simulink model "DS_SS"  (R2018a)
settings: Solver=ode4  StartTime=0.0  StopTime=N*Tb  FixedStep=Tsampling  RelTol=1e-9
values from neighbouring files (symbols this model uses):
  Eb = 2    [DS_Script.m]
  FrecSignal = MultFrec*(1/Tc)    [DS_MultUs_Script.m]    (also in DS_Script.m = 7500)
  Tb = 1/100    (= 0.01)    [DS_Script.m]
  Tc = Tb_min/(MultPer*Nchips)    [DS_MultUs_Script.m]    (also in DS_Script.m = 0.000666666666667)
libraries: commdigbbndpm3 x6, commseqgen3 x6, dspsigops x3, commutil2 x3, commrandsrc3 x3
settings Model: Creator=lukit  LastModifiedBy=geroo
settings DebuggingCC: LibraryContextMissingDiagnostic=warning
settings SFSimCC: SimUseLocalCustomCode=on
settings RTWCC: RTWUseLocalCustomCode=on

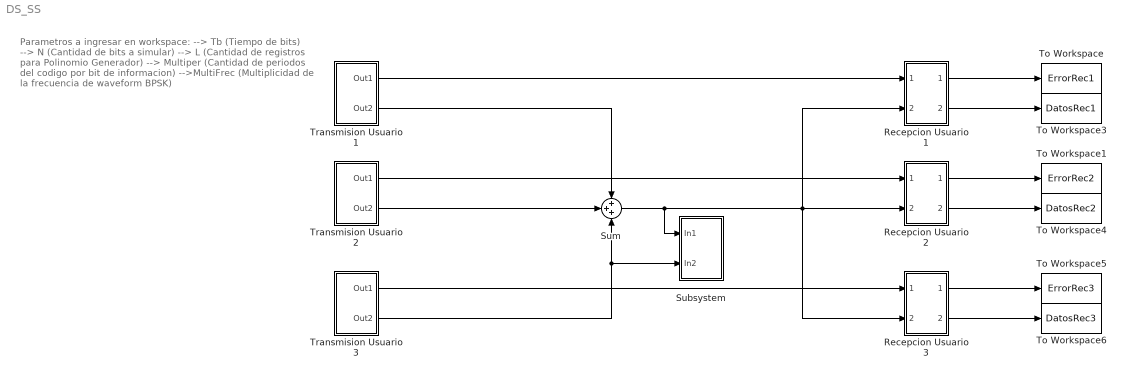
== system DS_SS ==
  note: Parametros a ingresar en workspace:
      | --> Tb (Tiempo de bits)
      | --> N  (Cantidad de bits a simular)
      | --> L   (Cantidad de registros para Polinomio Generador)
      | --> Multiper  (Cantidad de periodos del codigo por bit de informacion)
      | -->MultiFrec (Multiplicidad de la frecuencia de waveform BPSK)
  "Recepcion Usuario 1 " : Subsystem
  "Recepcion Usuario 2 " : Subsystem
  Recepcion Usuario 3 : Subsystem
  Subsystem : Subsystem
  Sum : Sum  Inputs=+++
  To Workspace : ToWorkspace  VariableName=ErrorRec1  SampleTime=-1
      settings: Save2DSignal=2-D array (concatenate along first dimension)
  To Workspace1 : ToWorkspace  VariableName=ErrorRec2  SampleTime=-1
      settings: Save2DSignal=2-D array (concatenate along first dimension)
  To Workspace3 : ToWorkspace  VariableName=DatosRec1  SampleTime=-1
      settings: Save2DSignal=2-D array (concatenate along first dimension)
  To Workspace4 : ToWorkspace  VariableName=DatosRec2  SampleTime=-1
      settings: Save2DSignal=2-D array (concatenate along first dimension)
  To Workspace5 : ToWorkspace  VariableName=ErrorRec3  SampleTime=-1
      settings: Save2DSignal=2-D array (concatenate along first dimension)
  To Workspace6 : ToWorkspace  VariableName=DatosRec3  SampleTime=-1
      settings: Save2DSignal=2-D array (concatenate along first dimension)
  "Transmision Usuario 1 " : Subsystem
  "Transmision Usuario 2 " : Subsystem
  "Transmision Usuario 3 " : Subsystem
  wires:
  "Transmision Usuario 1 "/1(Out1) -> "Recepcion Usuario 1 "/1(In1)
  "Transmision Usuario 2 "/1(Out1) -> "Recepcion Usuario 2 "/1(In1)
  "Transmision Usuario 3 "/1(Out1) -> Recepcion Usuario 3/1(In1)
  Sum/1 -> Subsystem/1(In1), Recepcion Usuario 3/2(In2), "Recepcion Usuario 1 "/2(In2), "Recepcion Usuario 2 "/2(In2)
  "Transmision Usuario 2 "/2(Out2) -> Sum/2
  "Transmision Usuario 1 "/2(Out2) -> Sum/1
  "Transmision Usuario 3 "/2(Out2) -> Subsystem/2(In2), Sum/3
  "Recepcion Usuario 1 "/1(Out1) -> To Workspace/1
  "Recepcion Usuario 1 "/2(Out2) -> To Workspace3/1
  Recepcion Usuario 3/1(Out1) -> To Workspace5/1
  Recepcion Usuario 3/2(Out2) -> To Workspace6/1
  "Recepcion Usuario 2 "/1(Out1) -> To Workspace1/1
  "Recepcion Usuario 2 "/2(Out2) -> To Workspace4/1

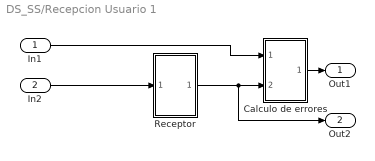
== system DS_SS/Recepcion Usuario 1  ==
  In1 : Inport
  In2 : Inport  Port=2
  Calculo de errores : Subsystem
  Receptor : Subsystem
  Out1 : Outport
  Out2 : Outport  Port=2
  wires:
  Calculo de errores/1(Out1) -> Out1/1
  In1/1 -> Calculo de errores/1(In1)
  Receptor/1(Out1) -> Out2/1, Calculo de errores/2(In2)
  In2/1 -> Receptor/1(In1)

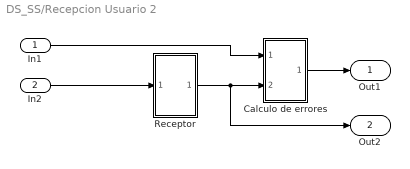
== system DS_SS/Recepcion Usuario 2  ==
  In1 : Inport
  In2 : Inport  Port=2
  Calculo de errores : Subsystem
  Receptor : Subsystem
  Out1 : Outport
  Out2 : Outport  Port=2
  wires:
  Calculo de errores/1(Out1) -> Out1/1
  In1/1 -> Calculo de errores/1(In1)
  Receptor/1(Out1) -> Out2/1, Calculo de errores/2(In2)
  In2/1 -> Receptor/1(In1)

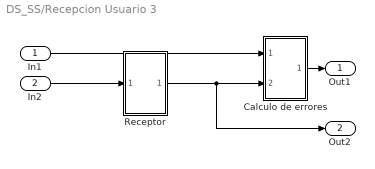
== system DS_SS/Recepcion Usuario 3 ==
  In1 : Inport
  In2 : Inport  Port=2
  "Calculo de errores " : Subsystem
  "Receptor " : Subsystem
  Out1 : Outport
  Out2 : Outport  Port=2
  wires:
  "Calculo de errores "/1(Out1) -> Out1/1
  In1/1 -> "Calculo de errores "/1(In1)
  "Receptor "/1(Out1) -> Out2/1, "Calculo de errores "/2(In2)
  In2/1 -> "Receptor "/1(In1)

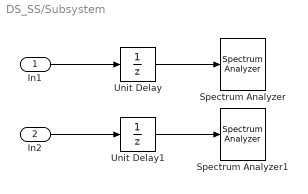
== system DS_SS/Subsystem ==
  In1 : Inport
  In2 : Inport  Port=2
  Spectrum Analyzer : SpectrumAnalyzer
  Spectrum Analyzer1 : SpectrumAnalyzer
  Unit Delay : UnitDelay  SampleTime=-1
  Unit Delay1 : UnitDelay  SampleTime=-1
  wires:
  Unit Delay/1 -> Spectrum Analyzer/1
  In1/1 -> Unit Delay/1
  In2/1 -> Unit Delay1/1
  Unit Delay1/1 -> Spectrum Analyzer1/1

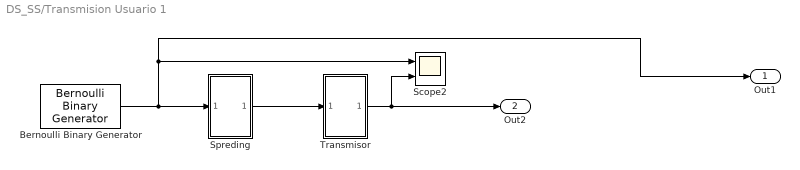
== system DS_SS/Transmision Usuario 1  ==
  Bernoulli Binary Generator : commrandsrc3/Bernoulli Binary Generator  ProbabilityOfZero=0.5  SeedSource=Auto  Seed=0  SampleTime=Tb  SamplesPerFrame=1  OutputDataType=double  SimulateUsing=Interpreted execution
  Scope2 : Scope  NumInputPorts=2
  "Spreding " : Subsystem
  Transmisor : Subsystem
  Out1 : Outport
  Out2 : Outport  Port=2
  wires:
  "Spreding "/1(Out1) -> Transmisor/1(In1)
  Bernoulli Binary Generator/1 -> Out1/1, Scope2/1, "Spreding "/1(In1)
  Transmisor/1(Out1) -> Out2/1, Scope2/2

== system DS_SS/Transmision Usuario 2  ==
  Bernoulli Binary Generator : commrandsrc3/Bernoulli Binary Generator  ProbabilityOfZero=0.5  SeedSource=Auto  Seed=0  SampleTime=Tb  SamplesPerFrame=1  OutputDataType=double  SimulateUsing=Interpreted execution
  Scope2 : Scope  NumInputPorts=2
  Spreding : Subsystem
  modulador BPSK : Subsystem
  Out1 : Outport
  Out2 : Outport  Port=2
  wires:
  Spreding/1(Out1) -> modulador BPSK/1(In1)
  Bernoulli Binary Generator/1 -> Out1/1, Scope2/1, Spreding/1(In1)
  modulador BPSK/1(Out1) -> Out2/1, Scope2/2

== system DS_SS/Transmision Usuario 3  ==
  Bernoulli Binary Generator : commrandsrc3/Bernoulli Binary Generator  ProbabilityOfZero=0.5  SeedSource=Auto  Seed=0  SampleTime=Tb  SamplesPerFrame=1  OutputDataType=double  SimulateUsing=Interpreted execution
  Scope2 : Scope  NumInputPorts=2
  "Spreding " : Subsystem
  modulador BPSK : Subsystem
  Out1 : Outport
  Out2 : Outport  Port=2
  wires:
  "Spreding "/1(Out1) -> modulador BPSK/1(In1)
  Bernoulli Binary Generator/1 -> Out1/1, Scope2/1, "Spreding "/1(In1)
  modulador BPSK/1(Out1) -> Out2/1, Scope2/2

== system DS_SS/Recepcion Usuario 1 /Calculo de errores ==
  In1 : Inport
  In2 : Inport  Port=2
  Scope4 : Scope  NumInputPorts=3
  Sum : Sum  Inputs=|+-
  Unit Delay : UnitDelay  SampleTime=-1
  Out1 : Outport
  wires:
  In2/1 -> Sum/2, Scope4/2
  Sum/1 -> Out1/1, Scope4/3
  Unit Delay/1 -> Scope4/1, Sum/1
  In1/1 -> Unit Delay/1

== system DS_SS/Recepcion Usuario 1 /Receptor ==
  In1 : Inport
  Demodulador BPSK : Subsystem
  Despreding : Subsystem
  Out1 : Outport
  wires:
  In1/1 -> Despreding/1(In1)
  Demodulador BPSK/1(Out1) -> Out1/1
  Despreding/1(Out1) -> Demodulador BPSK/1(In1)

== system DS_SS/Recepcion Usuario 2 /Calculo de errores ==
  In1 : Inport
  In2 : Inport  Port=2
  Scope4 : Scope  NumInputPorts=3
  Sum : Sum  Inputs=|+-
  Unit Delay : UnitDelay  SampleTime=-1
  Out1 : Outport
  wires:
  In2/1 -> Sum/2, Scope4/2
  Sum/1 -> Out1/1, Scope4/3
  Unit Delay/1 -> Scope4/1, Sum/1
  In1/1 -> Unit Delay/1

== system DS_SS/Recepcion Usuario 2 /Receptor ==
  In1 : Inport
  Demodulador Coherente : Subsystem
  "Despreding " : Subsystem
  Out1 : Outport
  wires:
  In1/1 -> "Despreding "/1(In1)
  "Despreding "/1(Out1) -> Demodulador Coherente/1(In1)
  Demodulador Coherente/1(Out1) -> Out1/1

== system DS_SS/Recepcion Usuario 3/Calculo de errores  ==
  In1 : Inport
  In2 : Inport  Port=2
  Scope4 : Scope  NumInputPorts=3
  Sum : Sum  Inputs=|+-
  Unit Delay : UnitDelay  SampleTime=-1
  Out1 : Outport
  wires:
  In2/1 -> Sum/2, Scope4/2
  Sum/1 -> Out1/1, Scope4/3
  Unit Delay/1 -> Scope4/1, Sum/1
  In1/1 -> Unit Delay/1

== system DS_SS/Recepcion Usuario 3/Receptor  ==
  In1 : Inport
  Demodulador BPSK : Subsystem
  Despreding : Subsystem
  Out1 : Outport
  wires:
  In1/1 -> Despreding/1(In1)
  Despreding/1(Out1) -> Demodulador BPSK/1(In1)
  Demodulador BPSK/1(Out1) -> Out1/1

== system DS_SS/Transmision Usuario 1 /Spreding  ==
  In1 : Inport
  PN Sequence Generator : commseqgen3/PN Sequence Generator  poly=PolGen  ini_sta=[0,0,0,1]  outBitMaskSource=Dialog parameter  shift=0  outVarSiz=off  maxOutSizeMode=Dialog parameter  maxOutSize=[10 1]  Ts=Tc  sampPerFrame=1  reset=off  bitPackedOutputs=off  outDataType=double  numPackedBits=8  bitPackDataSigned=off  bitPackedOutDType=double
      settings: SourceProductName=Communications System Toolbox
  Scope : Scope  NumInputPorts=3
  XOR : Logic  Operator=NXOR  IconShape=distinctive  AllPortsSameDT=off  OutDataTypeStr=boolean
  Out1 : Outport
  wires:
  PN Sequence Generator/1 -> Scope/2, XOR/2
  XOR/1 -> Scope/3, Out1/1
  In1/1 -> Scope/1, XOR/1

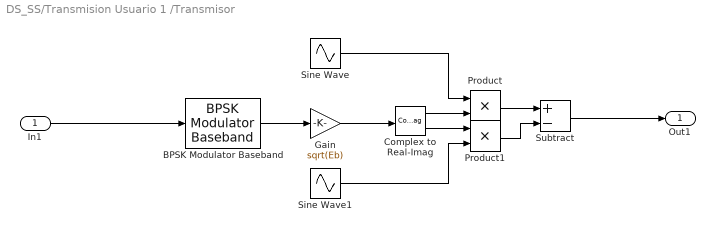
== system DS_SS/Transmision Usuario 1 /Transmisor ==
  In1 : Inport
  BPSK Modulator Baseband : commdigbbndpm3/BPSK Modulator Baseband  Ph=0  outDtype=double  outWordLen=16  outUDDataType=sfix(16)  outFracLenMode=Best precision  outFracLen=15  outDataTypeStr=double  outLastDataTypeStr=double
  Complex to Real-Imag : ComplexToRealImag
  Gain : Gain  Gain=sqrt(Eb)
  Product : Product
  Product1 : Product
  Sine Wave : Sin  Amplitude=sqrt(2/Tb)  Frequency=2*pi*FrecSignal  Phase=pi/2  SampleTime=0
  Sine Wave1 : Sin  Amplitude=sqrt(2/Tb)  Frequency=2*pi*FrecSignal  SampleTime=0
  Subtract : Sum  Inputs=+-
  Out1 : Outport
  wires:
  Sine Wave1/1 -> Product1/2
  Product1/1 -> Subtract/2
  BPSK Modulator Baseband/1 -> Gain/1
  Complex to Real-Imag/1 -> Product/2
  Sine Wave/1 -> Product/1
  Product/1 -> Subtract/1
  Subtract/1 -> Out1/1
  Complex to Real-Imag/2 -> Product1/1
  In1/1 -> BPSK Modulator Baseband/1
  Gain/1 -> Complex to Real-Imag/1

== system DS_SS/Transmision Usuario 2 /Spreding ==
  In1 : Inport
  PN Sequence Generator : commseqgen3/PN Sequence Generator  poly=PolGen  ini_sta=[1,1,1,1]  outBitMaskSource=Dialog parameter  shift=0  outVarSiz=off  maxOutSizeMode=Dialog parameter  maxOutSize=[10 1]  Ts=Tc  sampPerFrame=1  reset=off  bitPackedOutputs=off  outDataType=double  numPackedBits=8  bitPackDataSigned=off  bitPackedOutDType=double
      settings: SourceProductName=Communications System Toolbox
  Scope : Scope  NumInputPorts=3
  XOR : Logic  Operator=NXOR  IconShape=distinctive  AllPortsSameDT=off  OutDataTypeStr=boolean
  Out1 : Outport
  wires:
  PN Sequence Generator/1 -> Scope/2, XOR/2
  XOR/1 -> Scope/3, Out1/1
  In1/1 -> Scope/1, XOR/1

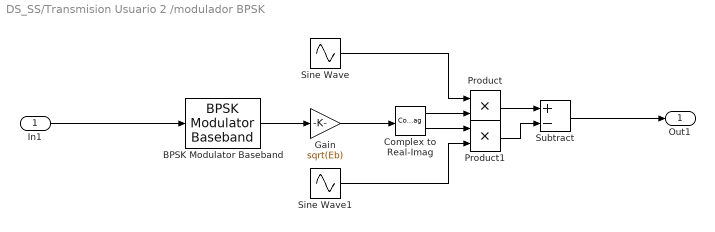
== system DS_SS/Transmision Usuario 2 /modulador BPSK ==
  In1 : Inport
  BPSK Modulator Baseband : commdigbbndpm3/BPSK Modulator Baseband  Ph=0  outDtype=double  outWordLen=16  outUDDataType=sfix(16)  outFracLenMode=Best precision  outFracLen=15  outDataTypeStr=double  outLastDataTypeStr=double
  Complex to Real-Imag : ComplexToRealImag
  Gain : Gain  Gain=sqrt(Eb)
  Product : Product
  Product1 : Product
  Sine Wave : Sin  Amplitude=sqrt(2/Tb)  Frequency=2*pi*FrecSignal  Phase=pi/2  SampleTime=0
  Sine Wave1 : Sin  Amplitude=sqrt(2/Tb)  Frequency=2*pi*FrecSignal  SampleTime=0
  Subtract : Sum  Inputs=+-
  Out1 : Outport
  wires:
  Sine Wave1/1 -> Product1/2
  Product1/1 -> Subtract/2
  BPSK Modulator Baseband/1 -> Gain/1
  Complex to Real-Imag/1 -> Product/2
  Sine Wave/1 -> Product/1
  Product/1 -> Subtract/1
  Subtract/1 -> Out1/1
  Complex to Real-Imag/2 -> Product1/1
  In1/1 -> BPSK Modulator Baseband/1
  Gain/1 -> Complex to Real-Imag/1

== system DS_SS/Transmision Usuario 3 /Spreding  ==
  In1 : Inport
  PN Sequence Generator : commseqgen3/PN Sequence Generator  poly=PolGen  ini_sta=[1,0,1,0]  outBitMaskSource=Dialog parameter  shift=0  outVarSiz=off  maxOutSizeMode=Dialog parameter  maxOutSize=[10 1]  Ts=Tc  sampPerFrame=1  reset=off  bitPackedOutputs=off  outDataType=double  numPackedBits=8  bitPackDataSigned=off  bitPackedOutDType=double
      settings: SourceProductName=Communications System Toolbox
  Scope : Scope  NumInputPorts=3
  XOR : Logic  Operator=NXOR  IconShape=distinctive  AllPortsSameDT=off  OutDataTypeStr=boolean
  Out1 : Outport
  wires:
  PN Sequence Generator/1 -> Scope/2, XOR/2
  XOR/1 -> Scope/3, Out1/1
  In1/1 -> Scope/1, XOR/1

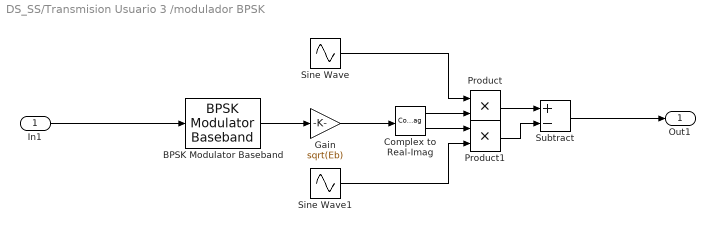
== system DS_SS/Transmision Usuario 3 /modulador BPSK ==
  In1 : Inport
  BPSK Modulator Baseband : commdigbbndpm3/BPSK Modulator Baseband  Ph=0  outDtype=double  outWordLen=16  outUDDataType=sfix(16)  outFracLenMode=Best precision  outFracLen=15  outDataTypeStr=double  outLastDataTypeStr=double
  Complex to Real-Imag : ComplexToRealImag
  Gain : Gain  Gain=sqrt(Eb)
  Product : Product
  Product1 : Product
  Sine Wave : Sin  Amplitude=sqrt(2/Tb)  Frequency=2*pi*FrecSignal  Phase=pi/2  SampleTime=0
  Sine Wave1 : Sin  Amplitude=sqrt(2/Tb)  Frequency=2*pi*FrecSignal  SampleTime=0
  Subtract : Sum  Inputs=+-
  Out1 : Outport
  wires:
  Sine Wave1/1 -> Product1/2
  Product1/1 -> Subtract/2
  BPSK Modulator Baseband/1 -> Gain/1
  Complex to Real-Imag/1 -> Product/2
  Sine Wave/1 -> Product/1
  Product/1 -> Subtract/1
  Subtract/1 -> Out1/1
  Complex to Real-Imag/2 -> Product1/1
  In1/1 -> BPSK Modulator Baseband/1
  Gain/1 -> Complex to Real-Imag/1

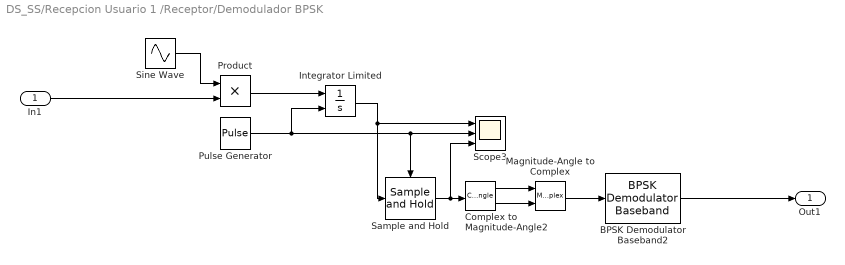
== system DS_SS/Recepcion Usuario 1 /Receptor/Demodulador BPSK ==
  In1 : Inport
  BPSK Demodulator Baseband2 : commdigbbndpm3/BPSK Demodulator Baseband  DecType=Hard decision  VarSource=Dialog  Variance=1  Ph=0  outDtype=Inherit via internal rule  derotateFactorWordLen=16  derotateFactorDataTypeStr=Inherit: Same word length as input  derotateFactorLastDataTypeStr=Inherit: Same word length as input
  Complex to Magnitude-Angle2 : ComplexToMagnitudeAngle
  Integrator Limited : Integrator  ExternalReset=rising  UpperSaturationLimit=1/2*1*(1/10)  LowerSaturationLimit=-1/2*1*(1/10)
  Magnitude-Angle to Complex : MagnitudeAngleToComplex
  Product : Product
  Pulse Generator : DiscretePulseGenerator  PulseType=Time based  Period=Tb  PulseWidth=99
  Sample and Hold : dspsigops/Sample and Hold  trig=Falling edge  initCond=0  latchinput=off
  Scope3 : Scope  NumInputPorts=3
  Sine Wave : Sin  Amplitude=sqrt(2/Tb)  Frequency=2*pi*FrecSignal  Phase=pi/2  SampleTime=0
  Out1 : Outport
  wires:
  Magnitude-Angle to Complex/1 -> BPSK Demodulator Baseband2/1
  Pulse Generator/1 -> Sample and Hold/Trigger, Scope3/2, Integrator Limited/2
  Complex to Magnitude-Angle2/2 -> Magnitude-Angle to Complex/2
  Product/1 -> Integrator Limited/1
  Complex to Magnitude-Angle2/1 -> Magnitude-Angle to Complex/1
  In1/1 -> Product/2
  Integrator Limited/1 -> Scope3/1, Sample and Hold/1
  Sample and Hold/1 -> Complex to Magnitude-Angle2/1, Scope3/3
  Sine Wave/1 -> Product/1
  BPSK Demodulator Baseband2/1 -> Out1/1

== system DS_SS/Recepcion Usuario 1 /Receptor/Despreding ==
  In1 : Inport
  PN Sequence Generator : commseqgen3/PN Sequence Generator  poly=PolGen  ini_sta=[0,0,0,1]  outBitMaskSource=Dialog parameter  shift=0  outVarSiz=off  maxOutSizeMode=Dialog parameter  maxOutSize=[10 1]  Ts=Tc  sampPerFrame=1  reset=off  bitPackedOutputs=off  outDataType=double  numPackedBits=8  bitPackDataSigned=off  bitPackedOutDType=double
      settings: SourceProductName=Communications System Toolbox
  Product1 : Product
  Scope : Scope  NumInputPorts=3
  Unipolar to Bipolar Converter : commutil2/Unipolar to Bipolar Converter  M=2  polarity=Positive  dataType=Inherit via internal rule
      settings: SourceProductName=Communications System Toolbox
  Out1 : Outport
  wires:
  PN Sequence Generator/1 -> Unipolar to Bipolar Converter/1
  In1/1 -> Scope/1, Product1/1
  Unipolar to Bipolar Converter/1 -> Scope/2, Product1/2
  Product1/1 -> Scope/3, Out1/1

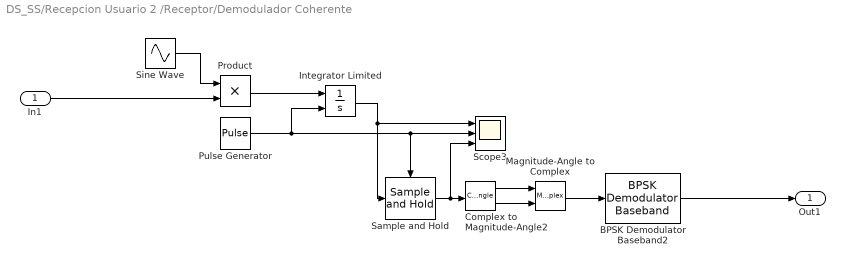
== system DS_SS/Recepcion Usuario 2 /Receptor/Demodulador Coherente ==
  In1 : Inport
  BPSK Demodulator Baseband2 : commdigbbndpm3/BPSK Demodulator Baseband  DecType=Hard decision  VarSource=Dialog  Variance=1  Ph=0  outDtype=Inherit via internal rule  derotateFactorWordLen=16  derotateFactorDataTypeStr=Inherit: Same word length as input  derotateFactorLastDataTypeStr=Inherit: Same word length as input
  Complex to Magnitude-Angle2 : ComplexToMagnitudeAngle
  Integrator Limited : Integrator  ExternalReset=rising  UpperSaturationLimit=1/2*1*(1/10)  LowerSaturationLimit=-1/2*1*(1/10)
  Magnitude-Angle to Complex : MagnitudeAngleToComplex
  Product : Product
  Pulse Generator : DiscretePulseGenerator  PulseType=Time based  Period=Tb  PulseWidth=99
  Sample and Hold : dspsigops/Sample and Hold  trig=Falling edge  initCond=0  latchinput=off
  Scope3 : Scope  NumInputPorts=3
  Sine Wave : Sin  Amplitude=sqrt(2/Tb)  Frequency=2*pi*FrecSignal  Phase=pi/2  SampleTime=0
  Out1 : Outport
  wires:
  Magnitude-Angle to Complex/1 -> BPSK Demodulator Baseband2/1
  Pulse Generator/1 -> Sample and Hold/Trigger, Scope3/2, Integrator Limited/2
  Complex to Magnitude-Angle2/2 -> Magnitude-Angle to Complex/2
  Product/1 -> Integrator Limited/1
  Complex to Magnitude-Angle2/1 -> Magnitude-Angle to Complex/1
  In1/1 -> Product/2
  Integrator Limited/1 -> Scope3/1, Sample and Hold/1
  Sample and Hold/1 -> Complex to Magnitude-Angle2/1, Scope3/3
  Sine Wave/1 -> Product/1
  BPSK Demodulator Baseband2/1 -> Out1/1

== system DS_SS/Recepcion Usuario 2 /Receptor/Despreding  ==
  In1 : Inport
  PN Sequence Generator : commseqgen3/PN Sequence Generator  poly=PolGen  ini_sta=[1,1,1,1]  outBitMaskSource=Dialog parameter  shift=0  outVarSiz=off  maxOutSizeMode=Dialog parameter  maxOutSize=[10 1]  Ts=Tc  sampPerFrame=1  reset=off  bitPackedOutputs=off  outDataType=double  numPackedBits=8  bitPackDataSigned=off  bitPackedOutDType=double
      settings: SourceProductName=Communications System Toolbox
  Product1 : Product
  Scope : Scope  NumInputPorts=3
  Unipolar to Bipolar Converter : commutil2/Unipolar to Bipolar Converter  M=2  polarity=Positive  dataType=Inherit via internal rule
      settings: SourceProductName=Communications System Toolbox
  Out1 : Outport
  wires:
  PN Sequence Generator/1 -> Unipolar to Bipolar Converter/1
  In1/1 -> Scope/1, Product1/1
  Unipolar to Bipolar Converter/1 -> Scope/2, Product1/2
  Product1/1 -> Scope/3, Out1/1

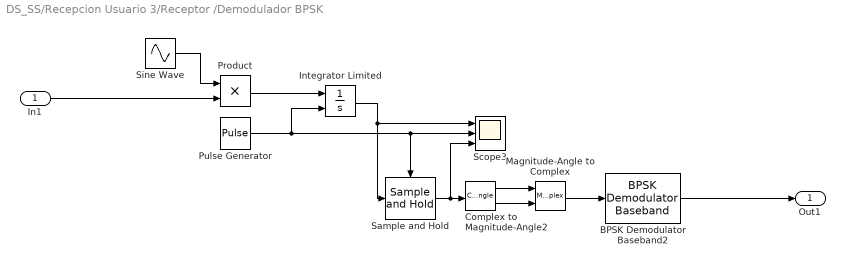
== system DS_SS/Recepcion Usuario 3/Receptor /Demodulador BPSK ==
  In1 : Inport
  BPSK Demodulator Baseband2 : commdigbbndpm3/BPSK Demodulator Baseband  DecType=Hard decision  VarSource=Dialog  Variance=1  Ph=0  outDtype=Inherit via internal rule  derotateFactorWordLen=16  derotateFactorDataTypeStr=Inherit: Same word length as input  derotateFactorLastDataTypeStr=Inherit: Same word length as input
  Complex to Magnitude-Angle2 : ComplexToMagnitudeAngle
  Integrator Limited : Integrator  ExternalReset=rising  UpperSaturationLimit=1/2*1*(1/10)  LowerSaturationLimit=-1/2*1*(1/10)
  Magnitude-Angle to Complex : MagnitudeAngleToComplex
  Product : Product
  Pulse Generator : DiscretePulseGenerator  PulseType=Time based  Period=Tb  PulseWidth=99
  Sample and Hold : dspsigops/Sample and Hold  trig=Falling edge  initCond=0  latchinput=off
  Scope3 : Scope  NumInputPorts=3
  Sine Wave : Sin  Amplitude=sqrt(2/Tb)  Frequency=2*pi*FrecSignal  Phase=pi/2  SampleTime=0
  Out1 : Outport
  wires:
  Magnitude-Angle to Complex/1 -> BPSK Demodulator Baseband2/1
  Pulse Generator/1 -> Sample and Hold/Trigger, Scope3/2, Integrator Limited/2
  Complex to Magnitude-Angle2/2 -> Magnitude-Angle to Complex/2
  Product/1 -> Integrator Limited/1
  Complex to Magnitude-Angle2/1 -> Magnitude-Angle to Complex/1
  In1/1 -> Product/2
  Integrator Limited/1 -> Scope3/1, Sample and Hold/1
  Sample and Hold/1 -> Complex to Magnitude-Angle2/1, Scope3/3
  Sine Wave/1 -> Product/1
  BPSK Demodulator Baseband2/1 -> Out1/1

== system DS_SS/Recepcion Usuario 3/Receptor /Despreding ==
  In1 : Inport
  PN Sequence Generator : commseqgen3/PN Sequence Generator  poly=PolGen  ini_sta=[1,0,1,0]  outBitMaskSource=Dialog parameter  shift=0  outVarSiz=off  maxOutSizeMode=Dialog parameter  maxOutSize=[10 1]  Ts=Tc  sampPerFrame=1  reset=off  bitPackedOutputs=off  outDataType=double  numPackedBits=8  bitPackDataSigned=off  bitPackedOutDType=double
      settings: SourceProductName=Communications System Toolbox
  Product1 : Product
  Scope : Scope  NumInputPorts=3
  Unipolar to Bipolar Converter : commutil2/Unipolar to Bipolar Converter  M=2  polarity=Positive  dataType=Inherit via internal rule
      settings: SourceProductName=Communications System Toolbox
  Out1 : Outport
  wires:
  PN Sequence Generator/1 -> Unipolar to Bipolar Converter/1
  In1/1 -> Scope/1, Product1/1
  Unipolar to Bipolar Converter/1 -> Scope/2, Product1/2
  Product1/1 -> Scope/3, Out1/1
